simulink model "OneOne_Conveyor"  (Simulink 8.1)
settings: Solver=ode45  StartTime=0.0  StopTime=9000.0  RelTol=1e-3
undefined symbols (not defined in the file or in its folder): rc_input, rc_LLC, rc_output, rc_sysAct
settings Model: Creator=obo  LastModifiedBy=zhangpn
settings DataIOCC: SignalLoggingSaveFormat=Dataset
settings OptimizationCC: ExpressionDepthLimit=128
settings DebuggingCC: UnderspecifiedInitializationDetection=Simplified  FcnCallInpInsideContextMsg=EnableAllAsError  StateNameClashWarn=none
settings GRTTargetCC: CodeReplacementLibrary=None  CombineOutputUpdateFcns=on  CPPClassGenCompliant=on  GRTInterface=off

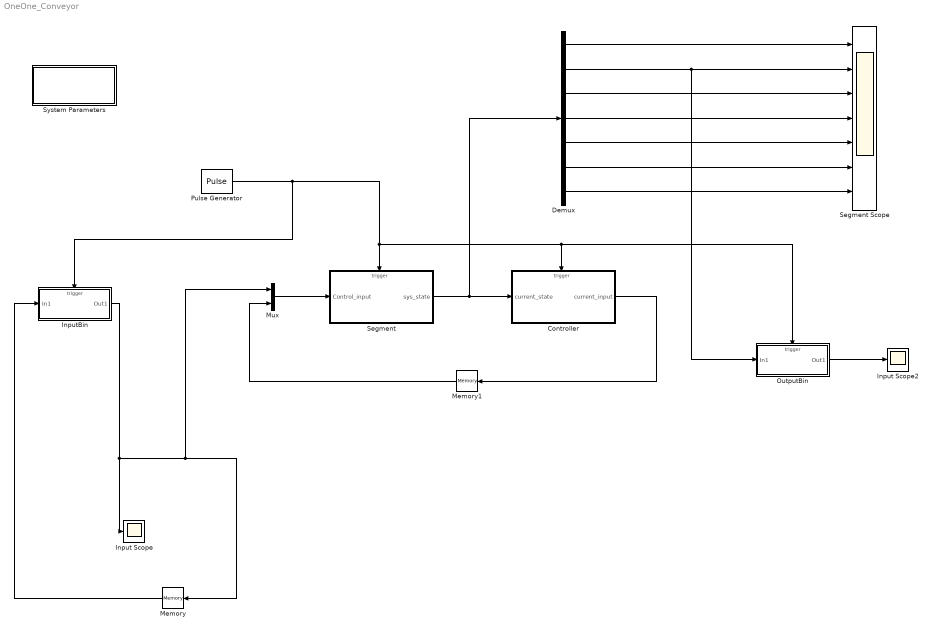
== system OneOne_Conveyor ==
  Controller : Subsystem  TreatAsAtomicUnit=on
  Demux : Demux  Outputs=7
  Input Scope : Scope
      settings: YMin=100  YMax=650
  Input Scope2 : Scope
      settings: TimeRange=9000  YMin=1.7e+06  YMax=3.7e+06  SaveName=ScopeData5
  InputBin : Subsystem
  Memory : Memory
  Memory1 : Memory
  Mux : Mux  Inputs=2
  OutputBin : Subsystem
  Pulse Generator : DiscretePulseGenerator  PulseType=Time based  Period=1  PulseWidth=50  PhaseDelay=0.01
  Segment : Subsystem  TreatAsAtomicUnit=on
  Segment Scope : Scope  NumInputPorts=7
      settings: TimeRange=9000  YMin=200~200~250~0~250~0.25~0.9  YMax=900~900~1000~500000~550~1~1  MaxDataPoints=10000
  System Parameters : Subsystem  mask(Initialization Block){}
      mask help: Calls sc_init.m on it's initialization to declare and initialize all global variables.
      mask init:
      | rc_init
      mask Display: disp('Initialization')
  wires:
  InputBin/1(Out1) -> Input Scope/1, Mux/1, Memory/1
  Memory/1 -> InputBin/1(In1)
  Segment/1(sys_state) -> Demux/1, Controller/1(current_state)
  Controller/1(current_input) -> Memory1/1
  Memory1/1 -> Mux/2
  Mux/1 -> Segment/1(Control_input)
  OutputBin/1(Out1) -> Input Scope2/1
  Demux/7 -> Segment Scope/7
  Demux/1 -> Segment Scope/1
  Demux/2 -> OutputBin/1(In1), Segment Scope/2
  Demux/3 -> Segment Scope/3
  Demux/4 -> Segment Scope/4
  Demux/5 -> Segment Scope/5
  Demux/6 -> Segment Scope/6
  ? -> ?
  Pulse Generator/1 -> InputBin/Trigger, OutputBin/Trigger, Controller/Trigger, Segment/Trigger

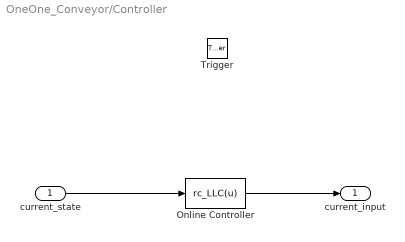
== system OneOne_Conveyor/Controller ==
  current_state : Inport
  Trigger : TriggerPort  TriggerType=falling  PortDimensions=1
  Online Controller : MATLABFcn  MATLABFcn=rc_LLC(u)  OutputDimensions=1  Output1D=off
  current_input : Outport  InitialOutput=0
  wires:
  Online Controller/1 -> current_input/1
  current_state/1 -> Online Controller/1

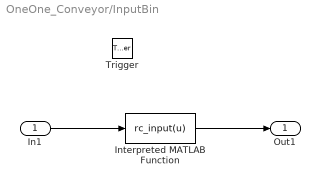
== system OneOne_Conveyor/InputBin ==
  In1 : Inport
  Trigger : TriggerPort  TriggerType=falling  PortDimensions=1
  Interpreted MATLAB Function : MATLABFcn  MATLABFcn=rc_input(u)  OutputDimensions=1
  Out1 : Outport  InitialOutput=[0]
  wires:
  In1/1 -> Interpreted MATLAB Function/1
  Interpreted MATLAB Function/1 -> Out1/1

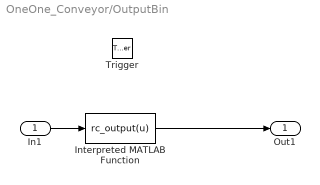
== system OneOne_Conveyor/OutputBin ==
  In1 : Inport
  Trigger : TriggerPort  TriggerType=falling  PortDimensions=1
  Interpreted MATLAB Function : MATLABFcn  MATLABFcn=rc_output(u)
  Out1 : Outport  InitialOutput=[0]
  wires:
  In1/1 -> Interpreted MATLAB Function/1
  Interpreted MATLAB Function/1 -> Out1/1

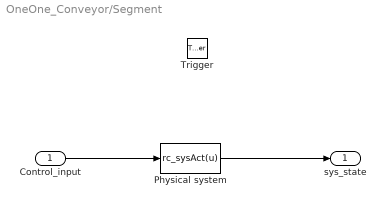
== system OneOne_Conveyor/Segment ==
  Control_input : Inport
  Trigger : TriggerPort  PortDimensions=1
  Physical system : MATLABFcn  MATLABFcn=rc_sysAct(u)  OutputDimensions=1*7  Output1D=off
  sys_state : Outport  InitialOutput=0
  wires:
  Control_input/1 -> Physical system/1
  Physical system/1 -> sys_state/1

== system OneOne_Conveyor/System Parameters ==
